simulink model "launcher"  (R2015b)
settings: Solver=VariableStepAuto  StartTime=0.0  StopTime=100000  RelTol=1e-3
settings Model: Creator=moormana  LastModifiedBy=moormana

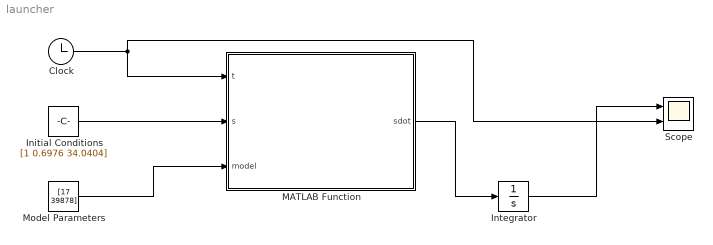
== system launcher ==
  Clock : Clock
  Initial Conditions : Constant  Value=[1 0.6976 34.0404]  VectorParams1D=off
  Integrator : Integrator
  MATLAB Function : MATLAB Function  TreatAsAtomicUnit=on
  Model Parameters : Constant  Value=[17 39878]  VectorParams1D=off
  Scope : Scope  NumInputPorts=2
  wires:
  Clock/1 -> Scope/2, MATLAB Function/1(t)
  Initial Conditions/1 -> MATLAB Function/2(s)
  Model Parameters/1 -> MATLAB Function/3(model)
  MATLAB Function/1(sdot) -> Integrator/1
  Integrator/1 -> Scope/1

== matlab function launcher/MATLAB Function ==
  data: t input; sdot output; s input; model input
function sdot   = lunardisk( t,s,model )
%UNTITLED Summary of this function goes here
%   Detailed explanation goes here

m   = model(1);
Izz = model(2);

sdot1 = s(2);
sdot2 = s(3)^2*s(1);
sdot3 =-2*m*s(1)*s(2)*s(3)/(Izz+m*s(1));

sdot = [sdot1 sdot2 sdot3]';
end
